simulink model "simulator_v1"  (R2022b)
settings: Solver=ode8  StartTime=0.0  StopTime=simulation_time  FixedStep=dt  RelTol=1e-3
libraries: aerolibanimutils x1, aerolibanim x1
settings Model: Creator=lasto  LastModifiedBy=lasto

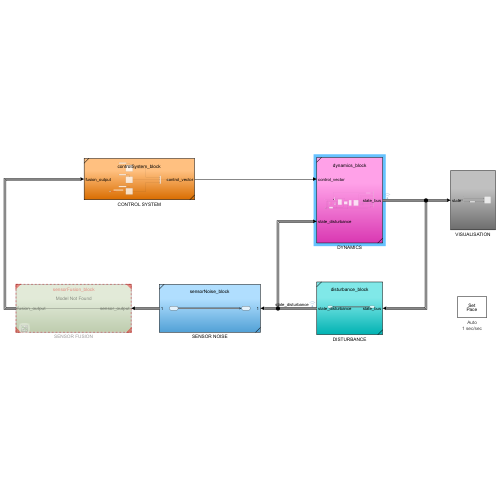
[thumbnail: Simulink's stored preview of the top-level diagram]
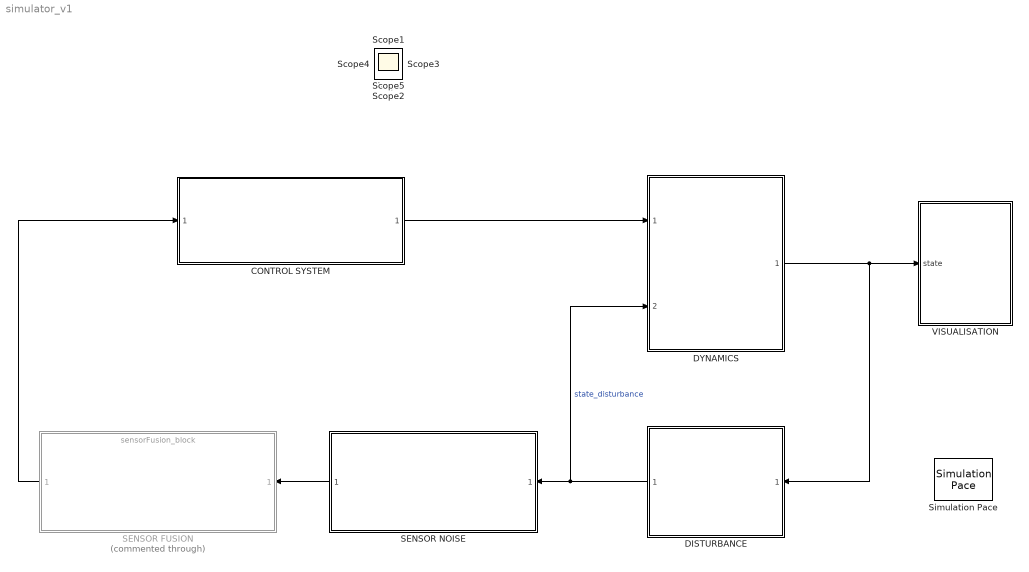
== system simulator_v1 ==
  CONTROL SYSTEM : Subsystem  ReferencedSubsystem=controlSystem_block
  DISTURBANCE : Subsystem  ReferencedSubsystem=disturbance_block
  DYNAMICS : Subsystem  ReferencedSubsystem=dynamics_block
  SENSOR FUSION : ModelReference  Commented=through  ModelNameDialog=sensorFusion_block.slx  SimulationMode=Normal  ModelReferenceVersion=1.7
  SENSOR NOISE : Subsystem  ReferencedSubsystem=sensorNoise_block
  Simulation Pace : aerolibanimutils/Simulation Pace  SimulationPace=1  SleepMode=Auto  OutputPaceError=off  SampleTime=-1
  VISUALISATION : Subsystem
  Scope{,1..5} (6 alike) : Scope
  wires:
  SENSOR NOISE/1 -> SENSOR FUSION/1
  DISTURBANCE/1 -> SENSOR NOISE/1, DYNAMICS/2  "state_disturbance"
  SENSOR FUSION/1 -> CONTROL SYSTEM/1
  CONTROL SYSTEM/1 -> DYNAMICS/1
  DYNAMICS/1 -> DISTURBANCE/1, VISUALISATION/1(state)

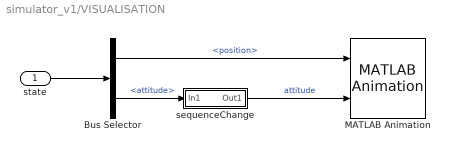
== system simulator_v1/VISUALISATION ==
  state : Inport
  Bus Selector : BusSelector  OutputSignals=position,attitude
  MATLAB Animation : aerolibanim/MATLAB Animation  Tag=Matlab Animation 6 DOF  Vehicles=1  Geometries='astredwedge.mat'  BoundingBoxCoordinates=[-50,50,-50,50,-50,50]  CameraOffset=[-150,-50,0]  CameraViewAngle=3  SampleTime=0.2  FigurePosition=[403,303,275,214]
  sequenceChange : Subsystem
  wires:
  Bus Selector/2 -> sequenceChange/1(In1)  "<attitude>"
  Bus Selector/1 -> MATLAB Animation/1  "<position>"
  state/1 -> Bus Selector/1
  sequenceChange/1(Out1) -> MATLAB Animation/2  "attitude"

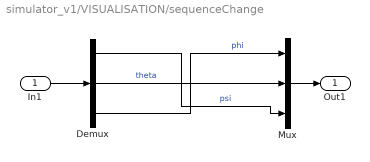
== system simulator_v1/VISUALISATION/sequenceChange ==
  In1 : Inport
  Demux : Demux  Outputs=3
  Mux : Mux  Inputs=3
  Out1 : Outport
  wires:
  In1/1 -> Demux/1
  Demux/3 -> Mux/1  "phi"
  Demux/2 -> Mux/2  "theta"
  Demux/1 -> Mux/3  "psi"
  Mux/1 -> Out1/1
